simulink model "ANFIS"  (R2015a)
settings: Solver=ode45  StartTime=0.02  StopTime=0.04  RelTol=1e-3
libraries: simulink x36, powerlib_meascontrol x30, powerlib x19, fuzblock x8
(part 2 of 2)

== system ANFIS/position controller3/Programmable Pulse Generator2 ==
  Amplitude : Inport
  Period : Inport  Port=2
  PulseWidth : Inport  Port=3
  PhaseDelay : Inport  Port=4
  Clock : Clock
  Constant : Constant  Value=1/100
  Constant1 : Constant  Value=0
  Data Type Conversion : DataTypeConversion  OutDataTypeStr=double
  Phase Delay Switch : Switch
  Product : Product  Inputs=3  RndMeth=Zero
  Product1 : Product  RndMeth=Zero
  Relational Operator : RelationalOperator  Operator=<=
  Sum2 : Sum  Inputs=+-
  mod : Math  Operator=mod  SaturateOnIntegerOverflow=on
  Pulse : Outport
  wires:
  Product/1 -> Relational Operator/2
  Product1/1 -> Pulse/1
  Data Type Conversion/1 -> Product1/2
  Relational Operator/1 -> Data Type Conversion/1
  Constant/1 -> Product/3
  PulseWidth/1 -> Product/2
  mod/1 -> Relational Operator/1
  Period/1 -> Product/1, mod/2
  Clock/1 -> Sum2/1
  PhaseDelay/1 -> Sum2/2
  Sum2/1 -> mod/1, Phase Delay Switch/2
  Amplitude/1 -> Phase Delay Switch/1
  Constant1/1 -> Phase Delay Switch/3
  Phase Delay Switch/1 -> Product1/1

== system ANFIS/position controller3/Programmable Pulse Generator3 ==
  Amplitude : Inport
  Period : Inport  Port=2
  PulseWidth : Inport  Port=3
  PhaseDelay : Inport  Port=4
  Clock : Clock
  Constant : Constant  Value=1/100
  Constant1 : Constant  Value=0
  Data Type Conversion : DataTypeConversion  OutDataTypeStr=double
  Phase Delay Switch : Switch
  Product : Product  Inputs=3  RndMeth=Zero
  Product1 : Product  RndMeth=Zero
  Relational Operator : RelationalOperator  Operator=<=
  Sum2 : Sum  Inputs=+-
  mod : Math  Operator=mod  SaturateOnIntegerOverflow=on
  Pulse : Outport
  wires:
  Phase Delay Switch/1 -> Product1/1
  Constant1/1 -> Phase Delay Switch/3
  Amplitude/1 -> Phase Delay Switch/1
  Sum2/1 -> Phase Delay Switch/2, mod/1
  PhaseDelay/1 -> Sum2/2
  Clock/1 -> Sum2/1
  Period/1 -> mod/2, Product/1
  mod/1 -> Relational Operator/1
  PulseWidth/1 -> Product/2
  Constant/1 -> Product/3
  Relational Operator/1 -> Data Type Conversion/1
  Data Type Conversion/1 -> Product1/2
  Product1/1 -> Pulse/1
  Product/1 -> Relational Operator/2

== system ANFIS/position controller3/Programmable Pulse Generator4 ==
  Amplitude : Inport
  Period : Inport  Port=2
  PulseWidth : Inport  Port=3
  PhaseDelay : Inport  Port=4
  Clock : Clock
  Constant : Constant  Value=1/100
  Constant1 : Constant  Value=0
  Data Type Conversion : DataTypeConversion  OutDataTypeStr=double
  Phase Delay Switch : Switch
  Product : Product  Inputs=3  RndMeth=Zero
  Product1 : Product  RndMeth=Zero
  Relational Operator : RelationalOperator  Operator=<=
  Sum2 : Sum  Inputs=+-
  mod : Math  Operator=mod  SaturateOnIntegerOverflow=on
  Pulse : Outport
  wires:
  Product/1 -> Relational Operator/2
  Product1/1 -> Pulse/1
  Data Type Conversion/1 -> Product1/2
  Relational Operator/1 -> Data Type Conversion/1
  Constant/1 -> Product/3
  PulseWidth/1 -> Product/2
  mod/1 -> Relational Operator/1
  Period/1 -> Product/1, mod/2
  Clock/1 -> Sum2/1
  PhaseDelay/1 -> Sum2/2
  Sum2/1 -> mod/1, Phase Delay Switch/2
  Amplitude/1 -> Phase Delay Switch/1
  Constant1/1 -> Phase Delay Switch/3
  Phase Delay Switch/1 -> Product1/1

== system ANFIS/position controller3/Programmable Pulse Generator5 ==
  Amplitude : Inport
  Period : Inport  Port=2
  PulseWidth : Inport  Port=3
  PhaseDelay : Inport  Port=4
  Clock : Clock
  Constant : Constant  Value=1/100
  Constant1 : Constant  Value=0
  Data Type Conversion : DataTypeConversion  OutDataTypeStr=double
  Phase Delay Switch : Switch
  Product : Product  Inputs=3  RndMeth=Zero
  Product1 : Product  RndMeth=Zero
  Relational Operator : RelationalOperator  Operator=<=
  Sum2 : Sum  Inputs=+-
  mod : Math  Operator=mod  SaturateOnIntegerOverflow=on
  Pulse : Outport
  wires:
  Phase Delay Switch/1 -> Product1/1
  Constant1/1 -> Phase Delay Switch/3
  Amplitude/1 -> Phase Delay Switch/1
  Sum2/1 -> Phase Delay Switch/2, mod/1
  PhaseDelay/1 -> Sum2/2
  Clock/1 -> Sum2/1
  Period/1 -> mod/2, Product/1
  mod/1 -> Relational Operator/1
  PulseWidth/1 -> Product/2
  Constant/1 -> Product/3
  Relational Operator/1 -> Data Type Conversion/1
  Data Type Conversion/1 -> Product1/2
  Product1/1 -> Pulse/1
  Product/1 -> Relational Operator/2

== system ANFIS/position controller3/Programmable Pulse Generator6 ==
  Amplitude : Inport
  Period : Inport  Port=2
  PulseWidth : Inport  Port=3
  PhaseDelay : Inport  Port=4
  Clock : Clock
  Constant : Constant  Value=1/100
  Constant1 : Constant  Value=0
  Data Type Conversion : DataTypeConversion  OutDataTypeStr=double
  Phase Delay Switch : Switch
  Product : Product  Inputs=3  RndMeth=Zero
  Product1 : Product  RndMeth=Zero
  Relational Operator : RelationalOperator  Operator=<=
  Sum2 : Sum  Inputs=+-
  mod : Math  Operator=mod  SaturateOnIntegerOverflow=on
  Pulse : Outport
  wires:
  Product/1 -> Relational Operator/2
  Product1/1 -> Pulse/1
  Data Type Conversion/1 -> Product1/2
  Relational Operator/1 -> Data Type Conversion/1
  Constant/1 -> Product/3
  PulseWidth/1 -> Product/2
  mod/1 -> Relational Operator/1
  Period/1 -> Product/1, mod/2
  Clock/1 -> Sum2/1
  PhaseDelay/1 -> Sum2/2
  Sum2/1 -> mod/1, Phase Delay Switch/2
  Amplitude/1 -> Phase Delay Switch/1
  Constant1/1 -> Phase Delay Switch/3
  Phase Delay Switch/1 -> Product1/1

== system ANFIS/position controller3/Programmable Pulse Generator7 ==
  Amplitude : Inport
  Period : Inport  Port=2
  PulseWidth : Inport  Port=3
  PhaseDelay : Inport  Port=4
  Clock : Clock
  Constant : Constant  Value=1/100
  Constant1 : Constant  Value=0
  Data Type Conversion : DataTypeConversion  OutDataTypeStr=double
  Phase Delay Switch : Switch
  Product : Product  Inputs=3  RndMeth=Zero
  Product1 : Product  RndMeth=Zero
  Relational Operator : RelationalOperator  Operator=<=
  Sum2 : Sum  Inputs=+-
  mod : Math  Operator=mod  SaturateOnIntegerOverflow=on
  Pulse : Outport
  wires:
  Phase Delay Switch/1 -> Product1/1
  Constant1/1 -> Phase Delay Switch/3
  Amplitude/1 -> Phase Delay Switch/1
  Sum2/1 -> Phase Delay Switch/2, mod/1
  PhaseDelay/1 -> Sum2/2
  Clock/1 -> Sum2/1
  Period/1 -> mod/2, Product/1
  mod/1 -> Relational Operator/1
  PulseWidth/1 -> Product/2
  Constant/1 -> Product/3
  Relational Operator/1 -> Data Type Conversion/1
  Data Type Conversion/1 -> Product1/2
  Product1/1 -> Pulse/1
  Product/1 -> Relational Operator/2

== system ANFIS/position controller3/Programmable Pulse Generator8 ==
  Amplitude : Inport
  Period : Inport  Port=2
  PulseWidth : Inport  Port=3
  PhaseDelay : Inport  Port=4
  Clock : Clock
  Constant : Constant  Value=1/100
  Constant1 : Constant  Value=0
  Data Type Conversion : DataTypeConversion  OutDataTypeStr=double
  Phase Delay Switch : Switch
  Product : Product  Inputs=3  RndMeth=Zero
  Product1 : Product  RndMeth=Zero
  Relational Operator : RelationalOperator  Operator=<=
  Sum2 : Sum  Inputs=+-
  mod : Math  Operator=mod  SaturateOnIntegerOverflow=on
  Pulse : Outport
  wires:
  Product/1 -> Relational Operator/2
  Product1/1 -> Pulse/1
  Data Type Conversion/1 -> Product1/2
  Relational Operator/1 -> Data Type Conversion/1
  Constant/1 -> Product/3
  PulseWidth/1 -> Product/2
  mod/1 -> Relational Operator/1
  Period/1 -> Product/1, mod/2
  Clock/1 -> Sum2/1
  PhaseDelay/1 -> Sum2/2
  Sum2/1 -> mod/1, Phase Delay Switch/2
  Amplitude/1 -> Phase Delay Switch/1
  Constant1/1 -> Phase Delay Switch/3
  Phase Delay Switch/1 -> Product1/1

== system ANFIS/position controller3/Programmable Pulse Generator9 ==
  Amplitude : Inport
  Period : Inport  Port=2
  PulseWidth : Inport  Port=3
  PhaseDelay : Inport  Port=4
  Clock : Clock
  Constant : Constant  Value=1/100
  Constant1 : Constant  Value=0
  Data Type Conversion : DataTypeConversion  OutDataTypeStr=double
  Phase Delay Switch : Switch
  Product : Product  Inputs=3  RndMeth=Zero
  Product1 : Product  RndMeth=Zero
  Relational Operator : RelationalOperator  Operator=<=
  Sum2 : Sum  Inputs=+-
  mod : Math  Operator=mod  SaturateOnIntegerOverflow=on
  Pulse : Outport
  wires:
  Phase Delay Switch/1 -> Product1/1
  Constant1/1 -> Phase Delay Switch/3
  Amplitude/1 -> Phase Delay Switch/1
  Sum2/1 -> Phase Delay Switch/2, mod/1
  PhaseDelay/1 -> Sum2/2
  Clock/1 -> Sum2/1
  Period/1 -> mod/2, Product/1
  mod/1 -> Relational Operator/1
  PulseWidth/1 -> Product/2
  Constant/1 -> Product/3
  Relational Operator/1 -> Data Type Conversion/1
  Data Type Conversion/1 -> Product1/2
  Product1/1 -> Pulse/1
  Product/1 -> Relational Operator/2

== matlab function ANFIS/MATLAB Function ==
  data: z1 input; y11 output; z2 input; z3 input; z4 input; z5 input; z6 input; z7 input; hal input; y12 output; y13 output; y14 output; y15 output; y21 output; y22 output; y23 output; y24 output; y25 output; y31 output; y32 output; y33 output; y34 output; y35 output
function [y11,y12,y13,y14,y15,y21,y22,...
    y23,y24,y25,y31,y32,y33,y34,y35]=...
    fcn(z1,z2,z3,z4,z5,z6,z7,hal)
%#codegen
z1 = z1/90;
z2 = z2/90;
z3 = z3/90;
z4 = z4/90;
z5 = z5/90;
z6 = z6/90;
z7 = z7/90;
y11 = 10;
        y12 = 10;
        y13 = 10;
        y14 = 10;
        y15 = 10;
        y21 = 10;
        y22 = 10;
        y23 = 10;
        y24 = 10;
        y25 = 10;
        y31 = 10;
        y32 = 10;
        y33 = 10;
        y34 = 10;
        y35 = 10;
z = round(hal);
switch z
    case 1
        y11 = z1;
        y12 = z2;
        y13 = z3;
        y14 = z4;
        y15 = z5;
        y21 = z6;
        y22 = 10;
        y23 = 10;
        y24 = 10;
        y25 = 10;
        y31 = z7;
        y32 = 10;
        y33 = 10;
        y34 = 10;
        y35 = 10;
    case 2
        y11 = z1;
        y12 = 10;
        y13 = 10;
        y14 = 10;
        y15 = 10;
        y21 = z2;
        y22 = z3;
        y23 = z4;
        y24 = z5;
        y25 = z6;
        y31 = z7;
        y32 = 10;
        y33 = 10;
        y34 = 10;
        y35 = 10;
    case 3
        y11 = z1;
        y12 = 10;
        y13 = 10;
        y14 = 10;
        y15 = 10;
        y21 = z2;
        y22 = 10;
        y23 = 10;
        y24 = 10;
        y25 = 10;
        y31 = z3;
        y32 = z4;
        y33 = z5;
        y34 = z6;
        y35 = z7;
    case 4
        y11 = z1;
        y12 = z2;
        y13 = z3;
        y14 = 10;
        y15 = 10;
        y21 = z4;
        y22 = z5;
        y23 = z6;
        y24 = 10;
        y25 = 10;
        y31 = z7;
        y32 = 10;
        y33 = 10;
        y34 = 10;
        y35 = 10;
    case 5
        y11 = z1;
        y12 = z2;
        y13 = z3;
        y14 = 10;
        y15 = 10;
        y21 = z4;
        y22 = 10;
        y23 = 10;
        y24 = 10;
        y25 = 10;
        y31 = z5;
        y32 = z6;
        y33 = z7;
        y34 = 10;
        y35 = 10;
    case 6 
        y11 = z1;
        y12 = 10;
        y13 = 10;
        y14 = 10;
        y15 = 10;
        y21 = z2;
        y22 = z3;
        y23 = z4;
        y24 = 10;
        y25 = 10;
        y31 = z5;
        y32 = z6;
        y33 = z7;
        y34 = 10;
        y35 = 10;
            
        
end
    
    
end
